simulink model "lazoCerradoAbierto"  (R2022a)
settings: Solver=VariableStepAuto  StartTime=0.0  StopTime=10.0  RelTol=1e-3
values from neighbouring files (symbols this model uses):
  A = 5    [smlk.m]
  den = [T,1]    [smlk.m]
  Kp = 1    [smlk.m]
  num = k    (= 0.75)    [smlk.m]
libraries: simulink x1
settings Model: Creator=Estudiantes  LastModifiedBy=Estudiantes

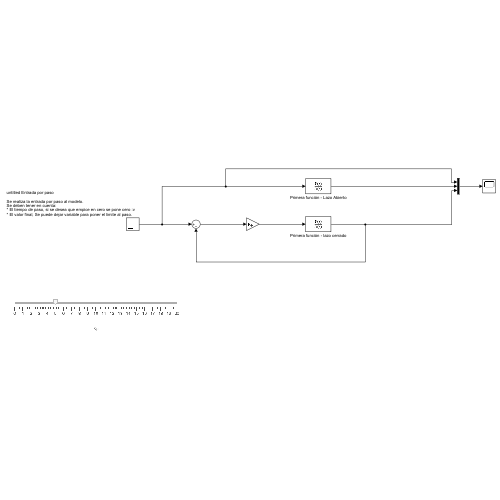
[thumbnail: Simulink's stored preview of the top-level diagram]
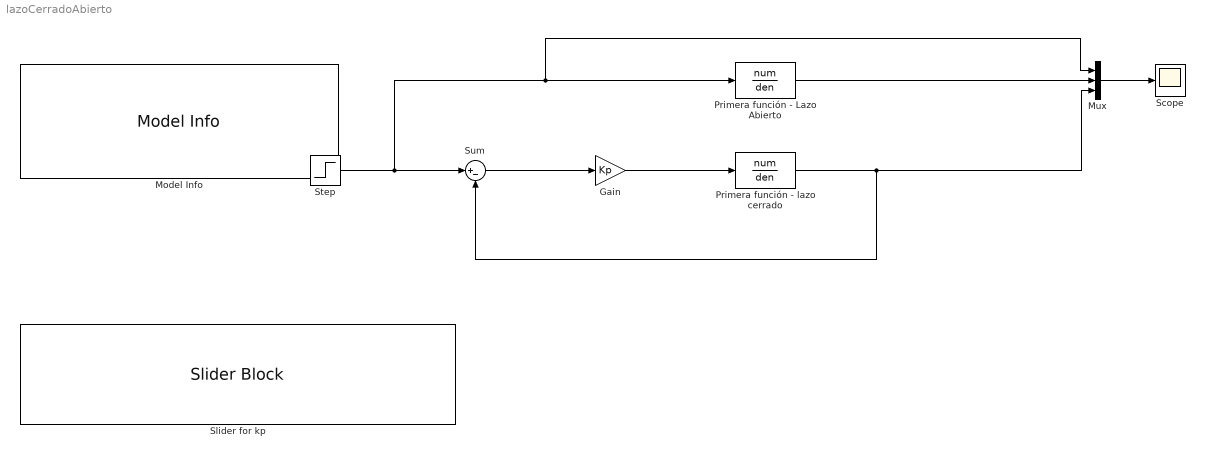
== system lazoCerradoAbierto ==
  Gain : Gain  Gain=Kp
  Model Info : simulink/Model-Wide Utilities/Model Info  Frame=off  DisplayStringWithTags=|  HorizontalTextAlignment=Left  LeftAlignmentValue=0.02
      | %<ModelName> Entrada por paso
      | %<Description> 
      | Se realiza la entrada por paso al modelo.
      | Se deben tener en cuenta:
      | * El tiempo de paso, si se desea que empice en cero se pone cero :v
      | * El valor final, Se puede dejar variable para poner el limite al paso.
  Mux : Mux  Inputs=3
  Primera función - Lazo Abierto : TransferFcn  Numerator=num  Denominator=den
  Primera función - lazo cerrado : TransferFcn  Numerator=num  Denominator=den
  Scope : Scope
  Slider for kp : SliderBlock  LabelPosition=Bottom  ScaleMax=20
  Step : Step  Time=0  After=A  SampleTime=0
  Sum : Sum  Inputs=|+-
  wires:
  Sum/1 -> Gain/1
  Gain/1 -> Primera función - lazo cerrado/1
  Primera función - lazo cerrado/1 -> Sum/2, Mux/3
  Step/1 -> Mux/1, Primera función - Lazo Abierto/1, Sum/1
  Primera función - Lazo Abierto/1 -> Mux/2
  Mux/1 -> Scope/1
